simulink model "gain_test_ElementWise"  (Simulink 9.0)
settings: Solver=ode3  StartTime=0.0  StopTime=10.0  FixedStep=0.100000  RelTol=1e-3  EnableMultiTasking=on
settings Model: SuppressorTable=22 serialization::archive 11 0 6 0 0 0 0 0  Creator=arnaud  LastModifiedBy=hbourbou
settings DataIOCC: LimitDataPoints=on  SaveFormat=Structure  SignalLoggingSaveFormat=ModelDataLogs
settings OptimizationCC: ExpressionDepthLimit=2147483647
settings DebuggingCC: SolverPrmCheckMsg=warning  UnnecessaryDatatypeConvMsg=warning  VectorMatrixConversionMsg=warning  FcnCallInpInsideContextMsg=warning  StateNameClashWarn=warning  StrictBusMsg=Warning
settings GRTTargetCC: CombineOutputUpdateFcns=off  GRTInterface=on

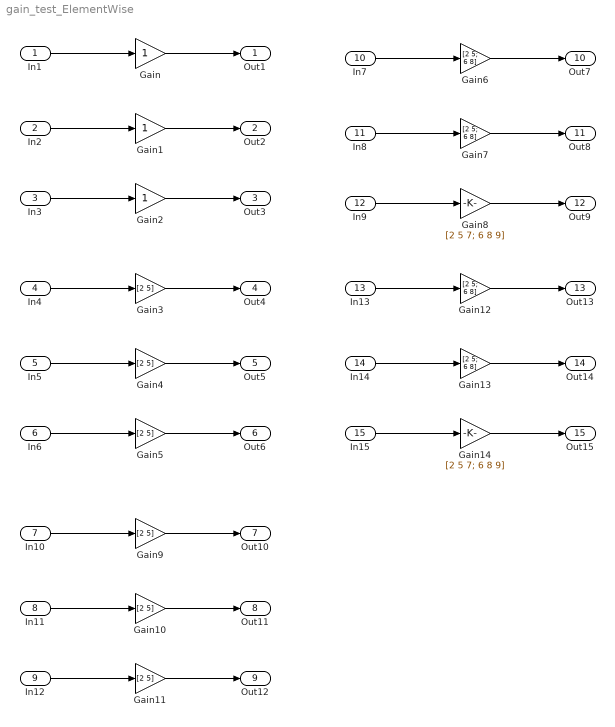
== system gain_test_ElementWise ==
  In1 : Inport  OutDataTypeStr=double
  In2 : Inport  Port=2  OutDataTypeStr=int8
  In3 : Inport  Port=3  OutDataTypeStr=boolean
  In4 : Inport  Port=4  OutDataTypeStr=double  PortDimensions=1
  In5 : Inport  Port=5  OutDataTypeStr=int8  PortDimensions=1
  In6 : Inport  Port=6  OutDataTypeStr=boolean  PortDimensions=1
  In10 : Inport  Port=7  OutDataTypeStr=double  PortDimensions=2
  In11 : Inport  Port=8  OutDataTypeStr=int8  PortDimensions=2
  In12 : Inport  Port=9  OutDataTypeStr=boolean  PortDimensions=2
  In7 : Inport  Port=10  OutDataTypeStr=double  PortDimensions=1
  In8 : Inport  Port=11  OutDataTypeStr=int8  PortDimensions=1
  In9 : Inport  Port=12  OutDataTypeStr=boolean  PortDimensions=1
  In13 : Inport  Port=13  OutDataTypeStr=double  PortDimensions=[2 2]
  In14 : Inport  Port=14  OutDataTypeStr=int8  PortDimensions=[2 2]
  In15 : Inport  Port=15  OutDataTypeStr=boolean  PortDimensions=[2 3]
  Gain : Gain
  Gain1 : Gain
  Gain{3..5,9..11} (6 alike) : Gain  Gain=[2 5]
  Gain{6..7,12..13} (4 alike) : Gain  Gain=[2 5; 6 8]
  Gain14 : Gain  Gain=[2 5 7; 6 8 9]
  Gain2 : Gain
  Gain8 : Gain  Gain=[2 5 7; 6 8 9]
  Out1 : Outport
  Out2 : Outport  Port=2
  Out3 : Outport  Port=3
  Out4 : Outport  Port=4
  Out5 : Outport  Port=5
  Out6 : Outport  Port=6
  Out10 : Outport  Port=7
  Out11 : Outport  Port=8
  Out12 : Outport  Port=9
  Out7 : Outport  Port=10
  Out8 : Outport  Port=11
  Out9 : Outport  Port=12
  Out13 : Outport  Port=13
  Out14 : Outport  Port=14
  Out15 : Outport  Port=15
  wires:
  In1/1 -> Gain/1
  Gain/1 -> Out1/1
  In2/1 -> Gain1/1
  Gain1/1 -> Out2/1
  In3/1 -> Gain2/1
  Gain2/1 -> Out3/1
  In4/1 -> Gain3/1
  Gain3/1 -> Out4/1
  In5/1 -> Gain4/1
  Gain4/1 -> Out5/1
  In6/1 -> Gain5/1
  Gain5/1 -> Out6/1
  In10/1 -> Gain9/1
  Gain9/1 -> Out10/1
  In11/1 -> Gain10/1
  Gain10/1 -> Out11/1
  In12/1 -> Gain11/1
  Gain11/1 -> Out12/1
  In7/1 -> Gain6/1
  Gain6/1 -> Out7/1
  In8/1 -> Gain7/1
  Gain7/1 -> Out8/1
  In9/1 -> Gain8/1
  Gain8/1 -> Out9/1
  In13/1 -> Gain12/1
  Gain12/1 -> Out13/1
  In14/1 -> Gain13/1
  Gain13/1 -> Out14/1
  In15/1 -> Gain14/1
  Gain14/1 -> Out15/1
